simulink library "SFCL"  (Simulink 7.7)
settings: Solver=ode45  StartTime=0.0  StopTime=10.0  RelTol=1e-3
undefined symbols (not defined in the file or in its folder): Fnom, Rshunt, Ta, Ts
libraries: SFCL x4, powerlib x2
Description:
  | /**
  |  * SFCL Simulink/SimPowerSystems implementation
  |  *
  |  * Copyright (c) 2011 Steven Blair
  |  *
  |  * Permission is hereby granted, free of charge, to any person obtaining a copy
  |  * of this software and associated documentation files (the "Software"), to deal
  |  * in the Software without restriction, including without limitation the rights
  |  * to use, copy, modify, merge, publish, distribute, sublicense, and/or sell
  |  * copies of the Software, and to permit persons to whom the Software is
  |  * furnished to do so, subject to the following conditions:
  |  *
  |  * The above copyright notice and this permission notice shall be included in
  |  * all copies or substantial portions of the Software.
  |  *
  |  * THE SOFTWARE IS PROVIDED "AS IS", WITHOUT WARRANTY OF ANY KIND, EXPRESS OR
  |  * IMPLIED, INCLUDING BUT NOT LIMITED TO THE WARRANTIES OF MERCHANTABILITY,
  |  * FITNESS FOR A PARTICULAR PURPOSE AND NONINFRINGEMENT. IN NO EVENT SHALL THE
  |  * AUTHORS OR COPYRIGHT HOLDERS BE LIABLE FOR ANY CLAIM, DAMAGES OR OTHER
  |  * LIABILITY, WHETHER IN AN ACTION OF CONTRACT, TORT OR OTHERWISE, ARISING FROM,
  |  * OUT OF OR IN CONNECTION WITH THE SOFTWARE OR THE USE OR OTHER DEALINGS IN
  |  * THE SOFTWARE.
  |  */
settings Model: Creator=Steven  LastModifiedBy=Steven

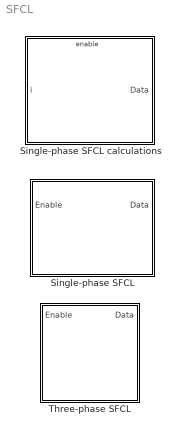
== system SFCL ==
  Single-phase SFCL : Subsystem  mask{Ta=Ta, Rshunt=Rshunt, Ts=Ts}
      mask prompts: Ta "Ambient temperature"; Rshunt "Shunt resistance"; Ts "Time step"
  Single-phase SFCL calculations : Subsystem  mask{Ta=Ta, Rshunt=Rshunt, Ts=Ts}
      mask prompts: Ta "Ambient temperature"; Rshunt "Shunt resistance"; Ts "Time step"
  Three-phase SFCL : Subsystem  mask{Ta=Ta, Rshunt=Rshunt, Ts=Ts}
      mask prompts: Ta "Ambient termperature"; Rshunt "Shunt resistance"; Ts "Time step"

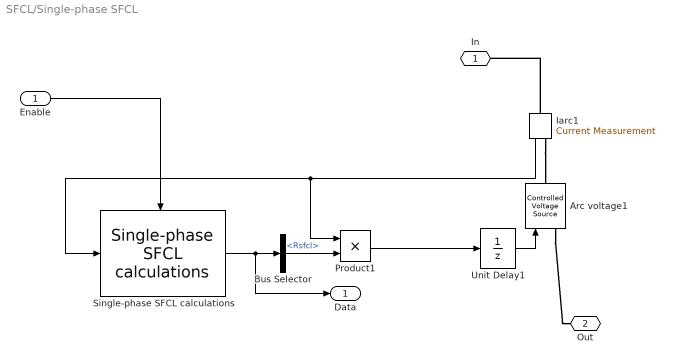
== system SFCL/Single-phase SFCL ==
  Enable : Inport
  Arc voltage1 : powerlib/Electrical Sources/Controlled Voltage Source  Description=source block  SystemSampleTime=-1  Initialize=on  Source_Type=AC  Amplitude=1e-6  Phase=0  Frequency=Fnom  Measurements=None
      settings: AttributesFormatString=\n
  Bus Selector : BusSelector  OutputSignals=Rsfcl
  Iarc1 : powerlib/Measurements/Current Measurement  Tag=PoWeRsYsTeMmEaSuReMeNt  SystemSampleTime=-1  PhasorSimulation=off  OutputType=Magnitude  PSBequivalent=0
  Product1 : Product  SaturateOnIntegerOverflow=on  InputSameDT=on  OutDataTypeStr=Inherit: Same as first input
  Single-phase SFCL calculations : SFCL/Single-phase SFCL calculations  SystemSampleTime=-1  Ta=Ta  Rshunt=Rshunt  Ts=Ts
  Unit Delay1 : UnitDelay  SampleTime=Ts
  In : PMIOPort  Port=1  Side=Left
  Out : PMIOPort  Port=2  Side=Right
  Data : Outport
  wires:
  Unit Delay1/1 -> Arc voltage1/1
  Product1/1 -> Unit Delay1/1
  Iarc1/1 -> Product1/1, Single-phase SFCL calculations/1
  Single-phase SFCL calculations/1 -> Bus Selector/1, Data/1
  Bus Selector/1 -> Product1/2  "<Rsfcl>"
  Enable/1 -> Single-phase SFCL calculations/Enable
  connections:
  Arc voltage1/LConn1 -- Out/RConn1
  Iarc1/RConn1 -- Arc voltage1/RConn1
  Iarc1/LConn1 -- In/RConn1

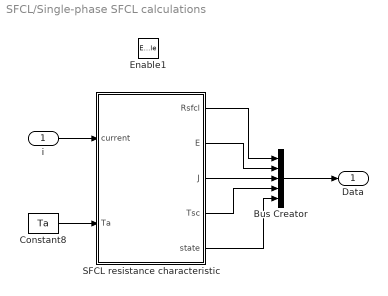
== system SFCL/Single-phase SFCL calculations ==
  i : Inport
  Enable1 : EnablePort
  Bus Creator : BusCreator  Inputs=5
  Constant8 : Constant  Value=Ta
  SFCL resistance characteristic : Stateflow chart  TreatAsAtomicUnit=on
  Data : Outport
  wires:
  i/1 -> SFCL resistance characteristic/1(current)
  SFCL resistance characteristic/1(Rsfcl) -> Bus Creator/1
  SFCL resistance characteristic/2(E) -> Bus Creator/2
  SFCL resistance characteristic/3(J) -> Bus Creator/3
  SFCL resistance characteristic/4(Tsc) -> Bus Creator/4
  SFCL resistance characteristic/5(state) -> Bus Creator/5
  Bus Creator/1 -> Data/1
  Constant8/1 -> SFCL resistance characteristic/2(Ta)

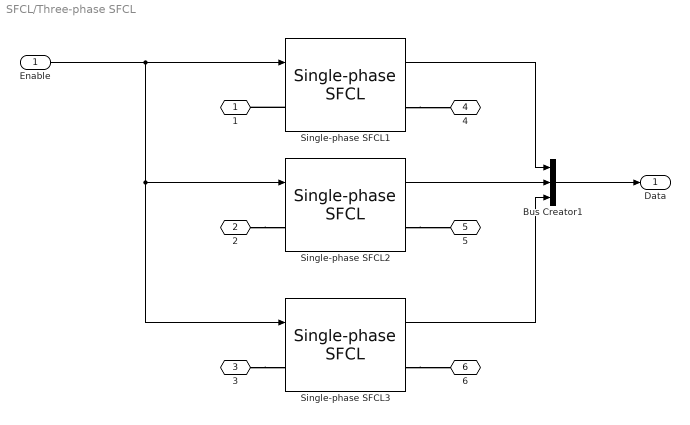
== system SFCL/Three-phase SFCL ==
  Enable : Inport
  Bus Creator1 : BusCreator  Inputs=3
  Single-phase SFCL1 : SFCL/Single-phase SFCL  SystemSampleTime=-1  Ta=Ta  Rshunt=Rshunt  Ts=Ts
  Single-phase SFCL2 : SFCL/Single-phase SFCL  SystemSampleTime=-1  Ta=Ta  Rshunt=Rshunt  Ts=Ts
  Single-phase SFCL3 : SFCL/Single-phase SFCL  SystemSampleTime=-1  Ta=Ta  Rshunt=Rshunt  Ts=Ts
  1 : PMIOPort  Port=1  Side=Left
  2 : PMIOPort  Port=2  Side=Left
  3 : PMIOPort  Port=3  Side=Left
  4 : PMIOPort  Port=4  Side=Right
  5 : PMIOPort  Port=5  Side=Right
  6 : PMIOPort  Port=6  Side=Right
  Data : Outport
  wires:
  Enable/1 -> Single-phase SFCL2/1, Single-phase SFCL3/1, Single-phase SFCL1/1
  Single-phase SFCL1/1 -> Bus Creator1/1
  Single-phase SFCL2/1 -> Bus Creator1/2
  Single-phase SFCL3/1 -> Bus Creator1/3
  Bus Creator1/1 -> Data/1
  connections:
  Single-phase SFCL1/LConn1 -- 1/RConn1
  Single-phase SFCL1/RConn1 -- 4/RConn1
  3/RConn1 -- Single-phase SFCL3/LConn1
  2/RConn1 -- Single-phase SFCL2/LConn1
  Single-phase SFCL2/RConn1 -- 5/RConn1
  Single-phase SFCL3/RConn1 -- 6/RConn1

== matlab function Single-phase SFCL calculations/SFCL resistance characteristic ==
  data: Rsfcl output double; E output double; J output double; current input double; Ta input double; Ts parameter double; Tsc output double; state output double
function [Rsfcl, E, J, Tsc, state] = fcn(current, Ta, Ts)

% superconductor dimensions and thermal properties
sc_length = 50.0;
sc_diameter = 0.004;                            % superconductor diameter (m)
sc_area = pi * (sc_diameter / 2)^2;             % superconductor cross-sectional area (m^2)
Cv = 1.0e6;
k = 1.5e3;
Csc = sc_length * sc_area * Cv;
Rsc = 1 / (k * sc_length * sc_diameter * pi);   % includes the total surface area (minus the "ends")
%nominal_resistance = rho_Tc * sc_length / sc_area;  % SFCL resistance at temperature=Tc

% superconductor characteristics
Jc_77K=1.5e7;               % critical current density at 77K (A/m^2)
E0=0.1;                     % E-field for transition from superconducting state to flux-flow state (V/m)
Ec=1e-6 * 100;              % definition of E-field required for Jc (V/m)
alpha_77K=6.0;              % exponent value during superconducting state (dimensionless)
beta=3;                     % exponent value during flux-flow state (dimensionless)
Tc=95;                      % critical temperature (K)
rho_Tc=1.0e-6;              % superconductor resistivity at Tc (ohm-m^2)

% inputs from previous iterations
persistent T;               % the instantaneous temperature of the superconductor
persistent prevE;           % store the E-field value from the previous iteration
persistent RsfclNew;        % history of Rsfcl values for averaging
persistent Qremoved;
persistent Qsc;
persistent time;            % elapsed simulation time

if isempty(T)
    T = Ta;                 % Ta is the ambient temperature of the coolant; it is assumed that this does not change
end
if isempty(prevE)
    prevE = 0.0;
end
if isempty(time)
    time = 0.0;
end
if isempty(RsfclNew)
    RsfclNew = [1e-6 1e-6 1e-6 1e-6 1e-6 1e-6 1e-6 1e-6 1e-6 1e-6];
end
if isempty(Qremoved)
    Qremoved = 0.0;
end
if isempty(Qsc)
    Qsc = 0.0;
end

RATE_LIMITING = 0;              % set to 1 to enable
AVERAGING_FILTER = 0;           % a value >0 sets the number of samples used for the averaging filter; a value of 0 disables; max value is 10
time = time + 1;
TEMPERATURE_TIMESTEPS = 1;      % defines number of timesteps needed for each thermal calculation; value of 1 means every timestep


J = abs(current) / sc_area;     % inputs from power system

if T < Tc
    if (prevE < E0)
        % superconducting
        state = 0;
    else
        % flux-flow
        state = 1;
    end
    
    Jc = Jc_77K * ((Tc - T) / (Tc - 77));
else
    % normal conducting
    state = 2;
    
    Jc = Jc_77K;    % value of Jc does not matter if T >= Tc
end

alpha_alt = log10(E0 / Ec) / log10( (Jc_77K / Jc)^(1 - (1/beta)) * (E0 / Ec)^(1 / alpha_77K) );
alpha = max(beta, alpha_alt);

% todo: prevent state from changing every timestep
if state == 0
    % superconducting
    E=Ec * (J / Jc)^alpha;
elseif state == 1
    % flux-flow
    E=E0 * (Ec / E0)^(beta/alpha_77K) * (Jc_77K / Jc) * (J / Jc_77K)^beta;
else
    % normal conducting
    E=rho_Tc * (T / Tc) * J;
end

prevE = E;

RsfclNew = [0, RsfclNew(1), RsfclNew(2), RsfclNew(3), RsfclNew(4), RsfclNew(5), RsfclNew(6), RsfclNew(7), RsfclNew(8), RsfclNew(9)];    % todo: convert to array of any length

if abs(current) > 0
    RsfclNew(1) = E * sc_length / abs(current);
else
    RsfclNew(1) = RsfclNew(2);
end

if (RATE_LIMITING == 1)
    %rate limiting; hold Rsfcl value at max rate, if rate is outwith limit
    RATE_LIMIT = 1.5;
    RATE_COMPARE = RsfclNew(2);
    if RsfclNew(1) > RATE_LIMIT * RATE_COMPARE
        RsfclNew(1) = RATE_LIMIT * RATE_COMPARE;
    elseif RsfclNew(1) < RATE_COMPARE / RATE_LIMIT
        RsfclNew(1) = RATE_COMPARE / RATE_LIMIT;
    end
end

if (AVERAGING_FILTER > 0)
    RsfclNew(1) = mean(RsfclNew(1:AVERAGING_FILTER));     % help smooth-out variations in Rsfcl
end
Rsfcl = RsfclNew(1);

% assume that if the flux-flow resistance >= the equivalent normal state resitance, then the superconductor has quenched
if Rsfcl >= (rho_Tc * (T / Tc) * J * sc_length / abs(current))
    state = 2;
    Rsfcl = (rho_Tc * (T / Tc) * J * sc_length / abs(current));
end

%QscDiff = current^2 * RsfclNew(1) * Ts;
QscDiff = current^2 * Rsfcl * Ts;
QremovedDiff = ((T - Ta) / Rsc) * Ts;
Qsc = Qsc + QscDiff;
Qremoved = Qremoved + QremovedDiff;

if (mod(time, TEMPERATURE_TIMESTEPS) == 0)
    T = T + (Qsc - Qremoved) / Csc;         % slight difference from [Langston2005]: Ta replaced by T
    Qsc = 0.0;
    Qremoved = 0.0;
end

Tsc = T;
